simulink model "Microgrid_PV_WG_Bat_EV_j_22b"  (R2022b)
settings: Solver=VariableStepAuto  StartTime=0.0  StopTime=1  RelTol=1e-3
undefined symbols (not defined in the file or in its folder): Acid, Ion, Lead, Lithium
libraries: slpidlib x35, spsabctodq0Lib x23, spsSeriesRLCBranchLib x19, spsCurrentMeasurementLib x13, spsVoltageMeasurementLib x11, spsThreePhaseVIMeasurementLib x10, spsPLL3phLib x9, spsThreePhaseSeriesRLCBranchLib x9, spsPower3phInstantaneousLib x8, spsIGBTDiodeLib x8, spsUniversalBridgeLib x7, spsPWMGeneratorDCDCLib x6
(part 5 of 5)

== system Microgrid_PV_WG_Bat_EV_j_22b/DC//AC2/下垂控制/电压电流双闭环1 ==
  Vd_ref : Inport
  Vd : Inport  Port=2
  Vq_ref : Inport  Port=3
  Vq : Inport  Port=4
  Id : Inport  Port=5
  Iq : Inport  Port=6
  ILd : Inport  Port=7
  ILq : Inport  Port=8
  wt : Inport  Port=9
  Constant : Constant  Value=0
  Gain : Gain  Gain=2*pi*50*20e-6
  Gain1 : Gain  Gain=2*pi*50*20e-6
  Gain2 : Gain  Gain=2*pi*50
  Gain3 : Gain  Gain=2*pi*50
  L1 : Constant  Value=5e-3
  L2 : Constant  Value=5e-3
  Mux : Mux  Inputs=3
  PID Controller : slpidlib/PID Controller  Controller=PI  Form=Parallel  TimeDomain=Continuous-time  UseExternalTs=off  SampleTime=-1  IntegratorMethod=Forward Euler  FilterMethod=Forward Euler  ControllerParametersSource=internal  P=0.5  I=10  UseKiTs=off  D=0  N=100  UseFilter=on  TunerSelectOption=Transfer Function Based (PID Tuner App)  InitialConditionSource=internal  InitialConditionForIntegrator=0  InitialConditionForFilter=0  DifferentiatorICPrevScaledInput=0  ExternalReset=none  TrackingMode=off  Kt=1  LimitOutput=off  SatLimitsSource=internal  UpperSaturationLimit=inf  LowerSaturationLimit=-inf  LinearizeAsGain=on  AntiWindupMode=none  Kb=1  LimitIntegrator=off  UpperIntegratorSaturationLimit=inf  LowerIntegratorSaturationLimit=-inf  POutMin=[]  POutMax=[]  IOutMin=[]  IOutMax=[]  DOutMin=[]  DOutMax=[]  NOutMin=[]  NOutMax=[]  SumOutMin=[]  SumOutMax=[]  SaturationOutMin=[]  SaturationOutMax=[]  PParamMin=[]  PParamMax=[]  IParamMin=[]  IParamMax=[]  DParamMin=[]  DParamMax=[]  NParamMin=[]  NParamMax=[]  KbParamMin=[]  KbParamMax=[]  KtParamMin=[]  KtParamMax=[]  KbOutMin=[]  KbOutMax=[]  KtOutMin=[]  KtOutMax=[]  IntegratorOutMin=[]  IntegratorOutMax=[]  FilterOutMin=[]  FilterOutMax=[]  SumI1OutMin=[]  SumI1OutMax=[]  SumI2OutMin=[]  SumI2OutMax=[]  SumI3OutMin=[]  SumI3OutMax=[]  SumI4OutMin=[]  SumI4OutMax=[]  SumDOutMin=[]  SumDOutMax=[]  DifferentiatorOutMin=[]  DifferentiatorOutMax=[]  FilterDiffOutCoefMin=[]  FilterDiffOutCoefMax=[]  ReciprocalOutMin=[]  ReciprocalOutMax=[]  SumDenOutMin=[]  SumDenOutMax=[]  SumNumOutMin=[]  SumNumOutMax=[]  DivideOutMin=[]  DivideOutMax=[]  UdiffTsProdOutMin=[]  UdiffTsProdOutMax=[]  NTsProdOutMin=[]  NTsProdOutMax=[]  UintegralTsProdOutMin=[]  UintegralTsProdOutMax=[]  UngainTsProdOutMin=[]  UngainTsProdOutMax=[]  IntegratorContinuousStateAttributes=''  IntegratorStateMustResolveToSignalObject=off  IntegratorRTWStateStorageClass=Auto  FilterContinuousStateAttributes=''  FilterStateMustResolveToSignalObject=off  FilterRTWStateStorageClass=Auto  ParallelPVariant=InternalParameters  IdealPVariant=Disabled  IVariant=InternalParameters  DVariant=Disabled  IntegratorVariant=Continuous  SatVariant=Disabled  AWVariant=Passthrough  PCopyVariant=Disabled  TRVariant=Disabled  FdbkBlocksVariant=Forward  IdealPFdbkVariant=Disabled  SatFdbkVariant=Disabled  DerivativeFilterVariant=Disabled  NVariant=Disabled  NCopyVariant=Disabled_SignalSpec  FilterICVariant=Disabled  IntegratorICVariant=InternalICs  ExternalResetVariant=Disabled  TRSumVariant=Passthrough  SumFdbkVariant=Disabled  SumVariant=Sum_PI  TsampFilterVariant=InternalTs  TsampNgainVariant=Passthrough  TsampIntegralVariant=Disabled_SignalSpec  ExternalSaturationOutDataTypeStr=Inherit: Same as second input
  PID Controller1 : slpidlib/PID Controller  Controller=PI  Form=Parallel  TimeDomain=Continuous-time  UseExternalTs=off  SampleTime=-1  IntegratorMethod=Forward Euler  FilterMethod=Forward Euler  ControllerParametersSource=internal  P=0.5  I=10  UseKiTs=off  D=0  N=100  UseFilter=on  TunerSelectOption=Transfer Function Based (PID Tuner App)  InitialConditionSource=internal  InitialConditionForIntegrator=0  InitialConditionForFilter=0  DifferentiatorICPrevScaledInput=0  ExternalReset=none  TrackingMode=off  Kt=1  LimitOutput=off  SatLimitsSource=internal  UpperSaturationLimit=inf  LowerSaturationLimit=-inf  LinearizeAsGain=on  AntiWindupMode=none  Kb=1  LimitIntegrator=off  UpperIntegratorSaturationLimit=inf  LowerIntegratorSaturationLimit=-inf  POutMin=[]  POutMax=[]  IOutMin=[]  IOutMax=[]  DOutMin=[]  DOutMax=[]  NOutMin=[]  NOutMax=[]  SumOutMin=[]  SumOutMax=[]  SaturationOutMin=[]  SaturationOutMax=[]  PParamMin=[]  PParamMax=[]  IParamMin=[]  IParamMax=[]  DParamMin=[]  DParamMax=[]  NParamMin=[]  NParamMax=[]  KbParamMin=[]  KbParamMax=[]  KtParamMin=[]  KtParamMax=[]  KbOutMin=[]  KbOutMax=[]  KtOutMin=[]  KtOutMax=[]  IntegratorOutMin=[]  IntegratorOutMax=[]  FilterOutMin=[]  FilterOutMax=[]  SumI1OutMin=[]  SumI1OutMax=[]  SumI2OutMin=[]  SumI2OutMax=[]  SumI3OutMin=[]  SumI3OutMax=[]  SumI4OutMin=[]  SumI4OutMax=[]  SumDOutMin=[]  SumDOutMax=[]  DifferentiatorOutMin=[]  DifferentiatorOutMax=[]  FilterDiffOutCoefMin=[]  FilterDiffOutCoefMax=[]  ReciprocalOutMin=[]  ReciprocalOutMax=[]  SumDenOutMin=[]  SumDenOutMax=[]  SumNumOutMin=[]  SumNumOutMax=[]  DivideOutMin=[]  DivideOutMax=[]  UdiffTsProdOutMin=[]  UdiffTsProdOutMax=[]  NTsProdOutMin=[]  NTsProdOutMax=[]  UintegralTsProdOutMin=[]  UintegralTsProdOutMax=[]  UngainTsProdOutMin=[]  UngainTsProdOutMax=[]  IntegratorContinuousStateAttributes=''  IntegratorStateMustResolveToSignalObject=off  IntegratorRTWStateStorageClass=Auto  FilterContinuousStateAttributes=''  FilterStateMustResolveToSignalObject=off  FilterRTWStateStorageClass=Auto  ParallelPVariant=InternalParameters  IdealPVariant=Disabled  IVariant=InternalParameters  DVariant=Disabled  IntegratorVariant=Continuous  SatVariant=Disabled  AWVariant=Passthrough  PCopyVariant=Disabled  TRVariant=Disabled  FdbkBlocksVariant=Forward  IdealPFdbkVariant=Disabled  SatFdbkVariant=Disabled  DerivativeFilterVariant=Disabled  NVariant=Disabled  NCopyVariant=Disabled_SignalSpec  FilterICVariant=Disabled  IntegratorICVariant=InternalICs  ExternalResetVariant=Disabled  TRSumVariant=Passthrough  SumFdbkVariant=Disabled  SumVariant=Sum_PI  TsampFilterVariant=InternalTs  TsampNgainVariant=Passthrough  TsampIntegralVariant=Disabled_SignalSpec  ExternalSaturationOutDataTypeStr=Inherit: Same as second input
  PID Controller2 : slpidlib/PID Controller  Controller=PI  Form=Parallel  TimeDomain=Continuous-time  UseExternalTs=off  SampleTime=-1  IntegratorMethod=Forward Euler  FilterMethod=Forward Euler  ControllerParametersSource=internal  P=50  I=1000  UseKiTs=off  D=0  N=100  UseFilter=on  TunerSelectOption=Transfer Function Based (PID Tuner App)  InitialConditionSource=internal  InitialConditionForIntegrator=0  InitialConditionForFilter=0  DifferentiatorICPrevScaledInput=0  ExternalReset=none  TrackingMode=off  Kt=1  LimitOutput=off  SatLimitsSource=internal  UpperSaturationLimit=inf  LowerSaturationLimit=-inf  LinearizeAsGain=on  AntiWindupMode=none  Kb=1  LimitIntegrator=off  UpperIntegratorSaturationLimit=inf  LowerIntegratorSaturationLimit=-inf  POutMin=[]  POutMax=[]  IOutMin=[]  IOutMax=[]  DOutMin=[]  DOutMax=[]  NOutMin=[]  NOutMax=[]  SumOutMin=[]  SumOutMax=[]  SaturationOutMin=[]  SaturationOutMax=[]  PParamMin=[]  PParamMax=[]  IParamMin=[]  IParamMax=[]  DParamMin=[]  DParamMax=[]  NParamMin=[]  NParamMax=[]  KbParamMin=[]  KbParamMax=[]  KtParamMin=[]  KtParamMax=[]  KbOutMin=[]  KbOutMax=[]  KtOutMin=[]  KtOutMax=[]  IntegratorOutMin=[]  IntegratorOutMax=[]  FilterOutMin=[]  FilterOutMax=[]  SumI1OutMin=[]  SumI1OutMax=[]  SumI2OutMin=[]  SumI2OutMax=[]  SumI3OutMin=[]  SumI3OutMax=[]  SumI4OutMin=[]  SumI4OutMax=[]  SumDOutMin=[]  SumDOutMax=[]  DifferentiatorOutMin=[]  DifferentiatorOutMax=[]  FilterDiffOutCoefMin=[]  FilterDiffOutCoefMax=[]  ReciprocalOutMin=[]  ReciprocalOutMax=[]  SumDenOutMin=[]  SumDenOutMax=[]  SumNumOutMin=[]  SumNumOutMax=[]  DivideOutMin=[]  DivideOutMax=[]  UdiffTsProdOutMin=[]  UdiffTsProdOutMax=[]  NTsProdOutMin=[]  NTsProdOutMax=[]  UintegralTsProdOutMin=[]  UintegralTsProdOutMax=[]  UngainTsProdOutMin=[]  UngainTsProdOutMax=[]  IntegratorContinuousStateAttributes=''  IntegratorStateMustResolveToSignalObject=off  IntegratorRTWStateStorageClass=Auto  FilterContinuousStateAttributes=''  FilterStateMustResolveToSignalObject=off  FilterRTWStateStorageClass=Auto  ParallelPVariant=InternalParameters  IdealPVariant=Disabled  IVariant=InternalParameters  DVariant=Disabled  IntegratorVariant=Continuous  SatVariant=Disabled  AWVariant=Passthrough  PCopyVariant=Disabled  TRVariant=Disabled  FdbkBlocksVariant=Forward  IdealPFdbkVariant=Disabled  SatFdbkVariant=Disabled  DerivativeFilterVariant=Disabled  NVariant=Disabled  NCopyVariant=Disabled_SignalSpec  FilterICVariant=Disabled  IntegratorICVariant=InternalICs  ExternalResetVariant=Disabled  TRSumVariant=Passthrough  SumFdbkVariant=Disabled  SumVariant=Sum_PI  TsampFilterVariant=InternalTs  TsampNgainVariant=Passthrough  TsampIntegralVariant=Disabled_SignalSpec  ExternalSaturationOutDataTypeStr=Inherit: Same as second input
  PID Controller3 : slpidlib/PID Controller  Controller=PI  Form=Parallel  TimeDomain=Continuous-time  UseExternalTs=off  SampleTime=-1  IntegratorMethod=Forward Euler  FilterMethod=Forward Euler  ControllerParametersSource=internal  P=50  I=1000  UseKiTs=off  D=0  N=100  UseFilter=on  TunerSelectOption=Transfer Function Based (PID Tuner App)  InitialConditionSource=internal  InitialConditionForIntegrator=0  InitialConditionForFilter=0  DifferentiatorICPrevScaledInput=0  ExternalReset=none  TrackingMode=off  Kt=1  LimitOutput=off  SatLimitsSource=internal  UpperSaturationLimit=inf  LowerSaturationLimit=-inf  LinearizeAsGain=on  AntiWindupMode=none  Kb=1  LimitIntegrator=off  UpperIntegratorSaturationLimit=inf  LowerIntegratorSaturationLimit=-inf  POutMin=[]  POutMax=[]  IOutMin=[]  IOutMax=[]  DOutMin=[]  DOutMax=[]  NOutMin=[]  NOutMax=[]  SumOutMin=[]  SumOutMax=[]  SaturationOutMin=[]  SaturationOutMax=[]  PParamMin=[]  PParamMax=[]  IParamMin=[]  IParamMax=[]  DParamMin=[]  DParamMax=[]  NParamMin=[]  NParamMax=[]  KbParamMin=[]  KbParamMax=[]  KtParamMin=[]  KtParamMax=[]  KbOutMin=[]  KbOutMax=[]  KtOutMin=[]  KtOutMax=[]  IntegratorOutMin=[]  IntegratorOutMax=[]  FilterOutMin=[]  FilterOutMax=[]  SumI1OutMin=[]  SumI1OutMax=[]  SumI2OutMin=[]  SumI2OutMax=[]  SumI3OutMin=[]  SumI3OutMax=[]  SumI4OutMin=[]  SumI4OutMax=[]  SumDOutMin=[]  SumDOutMax=[]  DifferentiatorOutMin=[]  DifferentiatorOutMax=[]  FilterDiffOutCoefMin=[]  FilterDiffOutCoefMax=[]  ReciprocalOutMin=[]  ReciprocalOutMax=[]  SumDenOutMin=[]  SumDenOutMax=[]  SumNumOutMin=[]  SumNumOutMax=[]  DivideOutMin=[]  DivideOutMax=[]  UdiffTsProdOutMin=[]  UdiffTsProdOutMax=[]  NTsProdOutMin=[]  NTsProdOutMax=[]  UintegralTsProdOutMin=[]  UintegralTsProdOutMax=[]  UngainTsProdOutMin=[]  UngainTsProdOutMax=[]  IntegratorContinuousStateAttributes=''  IntegratorStateMustResolveToSignalObject=off  IntegratorRTWStateStorageClass=Auto  FilterContinuousStateAttributes=''  FilterStateMustResolveToSignalObject=off  FilterRTWStateStorageClass=Auto  ParallelPVariant=InternalParameters  IdealPVariant=Disabled  IVariant=InternalParameters  DVariant=Disabled  IntegratorVariant=Continuous  SatVariant=Disabled  AWVariant=Passthrough  PCopyVariant=Disabled  TRVariant=Disabled  FdbkBlocksVariant=Forward  IdealPFdbkVariant=Disabled  SatFdbkVariant=Disabled  DerivativeFilterVariant=Disabled  NVariant=Disabled  NCopyVariant=Disabled_SignalSpec  FilterICVariant=Disabled  IntegratorICVariant=InternalICs  ExternalResetVariant=Disabled  TRSumVariant=Passthrough  SumFdbkVariant=Disabled  SumVariant=Sum_PI  TsampFilterVariant=InternalTs  TsampNgainVariant=Passthrough  TsampIntegralVariant=Disabled_SignalSpec  ExternalSaturationOutDataTypeStr=Inherit: Same as second input
  PWM Generator (2-Level) : spsPWMGenerator2LevelLib/PWM Generator (2-Level)  ModulatorType=Three-phase bridge (6 pulses)  ModulatorMode=Unsynchronized  Fc=10e3  Pc=90  nF=27  MinMax="[ -1  1 ]"  SamplingTechnique=Natural  ModulatingSignals=off  m=0.8  Freq=60  Phase=0  Ts=0  ShowCarrierOutport=off
  Product1 : Product
  Product2 : Product
  Sum : Sum  Inputs=|+-
  Sum1 : Sum  Inputs=-+|
  Sum2 : Sum  Inputs=++-
  Sum3 : Sum  Inputs=+++
  Sum4 : Sum  Inputs=|+-
  Sum5 : Sum  Inputs=-+|
  Sum6 : Sum  Inputs=++-
  Sum7 : Sum  Inputs=+++
  dq0 to abc : spsdq0toabcLib/dq0 to abc  Alignment=90 degrees behind phase A axis
  PWM : Outport
  wires:
  Vd_ref/1 -> Sum/1
  Vd/1 -> Sum6/1, Sum/2, Gain/1
  Sum/1 -> PID Controller/1
  Sum1/1 -> PID Controller1/1
  Vq/1 -> Sum7/3, Gain1/1, Sum1/1
  PID Controller/1 -> Sum2/2
  PID Controller1/1 -> Sum3/2
  Gain1/1 -> Sum2/3
  Id/1 -> Sum2/1
  Sum2/1 -> Sum4/1  "ILd_ref"
  Sum3/1 -> Sum5/2  "ILq_ref"
  ILd/1 -> Gain2/1, Sum4/2
  Sum4/1 -> PID Controller2/1
  Sum5/1 -> PID Controller3/1
  PID Controller2/1 -> Sum6/2
  PID Controller3/1 -> Sum7/2
  Gain2/1 -> Product2/1
  L2/1 -> Product2/2
  Gain/1 -> Sum3/1
  Iq/1 -> Sum3/3
  Vq_ref/1 -> Sum1/2
  Product2/1 -> Sum7/1
  L1/1 -> Product1/1
  Gain3/1 -> Product1/2
  ILq/1 -> Gain3/1, Sum5/1
  Product1/1 -> Sum6/3
  Sum6/1 -> Mux/1  "ILd_ref"
  Sum7/1 -> Mux/2  "ILq_ref"
  Constant/1 -> Mux/3
  Mux/1 -> dq0 to abc/1
  wt/1 -> dq0 to abc/2
  dq0 to abc/1 -> PWM Generator (2-Level)/1
  PWM Generator (2-Level)/1 -> PWM/1

== system Microgrid_PV_WG_Bat_EV_j_22b/Subsystem4/Subsystem2/Subsystem ==
  电流 : Inport
  Fcn : Fcn  Expr=60000*8.3145*(273+T)*N*u(1)/(2*96485*P*101325*Uf_H2/100*x/100)
  Saturation : Saturate  UpperLimit=inf  LowerLimit=1
  流速 : Outport
  wires:
  电流/1 -> Fcn/1
  Fcn/1 -> Saturation/1
  Saturation/1 -> 流速/1

== system Microgrid_PV_WG_Bat_EV_j_22b/Subsystem4/Subsystem2/Subsystem1 ==
  电流 : Inport
  Fcn : Fcn  Expr=60000*8.3145*(273+T)*N*u(1)/(2*96485*P*101325*Uf_H2/100*x/100)
  Saturation : Saturate  UpperLimit=inf  LowerLimit=1
  流速 : Outport
  wires:
  Saturation/1 -> 流速/1
  Fcn/1 -> Saturation/1
  电流/1 -> Fcn/1

== system Microgrid_PV_WG_Bat_EV_j_22b/Subsystem4/Subsystem2/Subsystem2 ==
  Vd : Inport
  Vq : Inport  Port=2
  P : Inport  Port=3
  Q : Inport  Port=4
  Add10 : Sum  Inputs=+-
  Add5 : Sum
  Add6 : Sum
  Divide2 : Product  Inputs=*/
  Divide3 : Product  Inputs=/*
  Gain4 : Gain  Gain=2/3
  Gain5 : Gain  Gain=2/3
  Product{7..12} (6 alike) : Product
  Id_ref : Outport
  Iq_ref : Outport  Port=2
  wires:
  Add6/1 -> Divide3/1, Divide2/2
  Vd/1 -> Product9/2, Product9/1, Product7/1, Product10/1
  Add10/1 -> Gain5/1
  Vq/1 -> Product12/1, Product8/1, Product11/2, Product11/1
  Product9/1 -> Add6/1
  Gain4/1 -> Divide2/1
  Product7/1 -> Add5/1
  P/1 -> Product12/2, Product7/2
  Product12/1 -> Add10/1
  Gain5/1 -> Divide3/2
  Add5/1 -> Gain4/1
  Product10/1 -> Add10/2
  Product8/1 -> Add5/2
  Product11/1 -> Add6/2
  Q/1 -> Product10/2, Product8/2
  Divide3/1 -> Iq_ref/1  "Iq_ref"
  Divide2/1 -> Id_ref/1  "Id_ref"

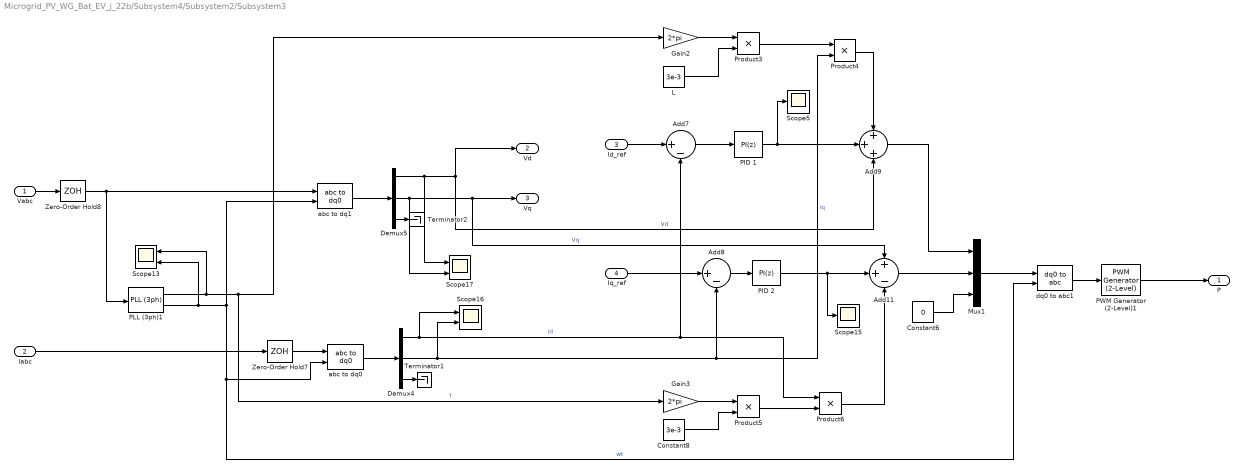
== system Microgrid_PV_WG_Bat_EV_j_22b/Subsystem4/Subsystem2/Subsystem3 ==
  Vabc : Inport
  Iabc : Inport  Port=2
  Id_ref : Inport  Port=3
  Iq_ref : Inport  Port=4
  Add11 : Sum  Inputs=++-
  Add7 : Sum  Inputs=|+-
  Add8 : Sum  Inputs=|+-
  Add9 : Sum  Inputs=+++
  Constant6 : Constant  Value=0
  Constant8 : Constant  Value=3e-3
  Demux4 : Demux  Outputs=3
  Demux5 : Demux  Outputs=3
  Gain2 : Gain  Gain=2*pi
  Gain3 : Gain  Gain=2*pi
  L : Constant  Value=3e-3
  Mux1 : Mux  Inputs=3
  PID 1 : slpidlib/PID Controller  Controller=PI  Form=Parallel  TimeDomain=Discrete-time  UseExternalTs=off  SampleTime=1e-5  IntegratorMethod=Forward Euler  FilterMethod=Forward Euler  ControllerParametersSource=internal  P=200  I=500  UseKiTs=off  D=0  N=100  UseFilter=on  TunerSelectOption=Transfer Function Based (PID Tuner App)  InitialConditionSource=internal  InitialConditionForIntegrator=0  InitialConditionForFilter=0  DifferentiatorICPrevScaledInput=0  ExternalReset=none  TrackingMode=off  Kt=1  LimitOutput=off  SatLimitsSource=internal  UpperSaturationLimit=0  LowerSaturationLimit=-860  LinearizeAsGain=on  AntiWindupMode=none  Kb=1  LimitIntegrator=off  UpperIntegratorSaturationLimit=inf  LowerIntegratorSaturationLimit=-inf  POutMin=[]  POutMax=[]  IOutMin=[]  IOutMax=[]  DOutMin=[]  DOutMax=[]  NOutMin=[]  NOutMax=[]  SumOutMin=[]  SumOutMax=[]  SaturationOutMin=[]  SaturationOutMax=[]  PParamMin=[]  PParamMax=[]  IParamMin=[]  IParamMax=[]  DParamMin=[]  DParamMax=[]  NParamMin=[]  NParamMax=[]  KbParamMin=[]  KbParamMax=[]  KtParamMin=[]  KtParamMax=[]  KbOutMin=[]  KbOutMax=[]  KtOutMin=[]  KtOutMax=[]  IntegratorOutMin=[]  IntegratorOutMax=[]  FilterOutMin=[]  FilterOutMax=[]  SumI1OutMin=[]  SumI1OutMax=[]  SumI2OutMin=[]  SumI2OutMax=[]  SumI3OutMin=[]  SumI3OutMax=[]  SumI4OutMin=[]  SumI4OutMax=[]  SumDOutMin=[]  SumDOutMax=[]  DifferentiatorOutMin=[]  DifferentiatorOutMax=[]  FilterDiffOutCoefMin=[]  FilterDiffOutCoefMax=[]  ReciprocalOutMin=[]  ReciprocalOutMax=[]  SumDenOutMin=[]  SumDenOutMax=[]  SumNumOutMin=[]  SumNumOutMax=[]  DivideOutMin=[]  DivideOutMax=[]  UdiffTsProdOutMin=[]  UdiffTsProdOutMax=[]  NTsProdOutMin=[]  NTsProdOutMax=[]  UintegralTsProdOutMin=[]  UintegralTsProdOutMax=[]  UngainTsProdOutMin=[]  UngainTsProdOutMax=[]  IntegratorContinuousStateAttributes=''  IntegratorStateMustResolveToSignalObject=off  IntegratorRTWStateStorageClass=Auto  FilterContinuousStateAttributes=''  FilterStateMustResolveToSignalObject=off  FilterRTWStateStorageClass=Auto  ParallelPVariant=InternalParameters  IdealPVariant=Disabled  IVariant=InternalParameters  DVariant=Disabled  IntegratorVariant=Discrete  SatVariant=Disabled  AWVariant=Passthrough  PCopyVariant=Disabled  TRVariant=Disabled  FdbkBlocksVariant=Forward  IdealPFdbkVariant=Disabled  SatFdbkVariant=Disabled  DerivativeFilterVariant=Disabled  NVariant=Disabled  NCopyVariant=Disabled_SignalSpec  FilterICVariant=Disabled  IntegratorICVariant=InternalICs  ExternalResetVariant=Disabled  TRSumVariant=Passthrough  SumFdbkVariant=Disabled  SumVariant=Sum_PI  TsampFilterVariant=InternalTs  TsampNgainVariant=Passthrough  TsampIntegralVariant=Disabled_SignalSpec  ExternalSaturationOutDataTypeStr=Inherit: Same as second input
  PID 2 : slpidlib/PID Controller  Controller=PI  Form=Parallel  TimeDomain=Discrete-time  UseExternalTs=off  SampleTime=1e-5  IntegratorMethod=Forward Euler  FilterMethod=Forward Euler  ControllerParametersSource=internal  P=200  I=500  UseKiTs=off  D=0  N=100  UseFilter=on  TunerSelectOption=Transfer Function Based (PID Tuner App)  InitialConditionSource=internal  InitialConditionForIntegrator=0  InitialConditionForFilter=0  DifferentiatorICPrevScaledInput=0  ExternalReset=none  TrackingMode=off  Kt=1  LimitOutput=off  SatLimitsSource=internal  UpperSaturationLimit=400  LowerSaturationLimit=-300  LinearizeAsGain=on  AntiWindupMode=none  Kb=1  LimitIntegrator=off  UpperIntegratorSaturationLimit=inf  LowerIntegratorSaturationLimit=-inf  POutMin=[]  POutMax=[]  IOutMin=[]  IOutMax=[]  DOutMin=[]  DOutMax=[]  NOutMin=[]  NOutMax=[]  SumOutMin=[]  SumOutMax=[]  SaturationOutMin=[]  SaturationOutMax=[]  PParamMin=[]  PParamMax=[]  IParamMin=[]  IParamMax=[]  DParamMin=[]  DParamMax=[]  NParamMin=[]  NParamMax=[]  KbParamMin=[]  KbParamMax=[]  KtParamMin=[]  KtParamMax=[]  KbOutMin=[]  KbOutMax=[]  KtOutMin=[]  KtOutMax=[]  IntegratorOutMin=[]  IntegratorOutMax=[]  FilterOutMin=[]  FilterOutMax=[]  SumI1OutMin=[]  SumI1OutMax=[]  SumI2OutMin=[]  SumI2OutMax=[]  SumI3OutMin=[]  SumI3OutMax=[]  SumI4OutMin=[]  SumI4OutMax=[]  SumDOutMin=[]  SumDOutMax=[]  DifferentiatorOutMin=[]  DifferentiatorOutMax=[]  FilterDiffOutCoefMin=[]  FilterDiffOutCoefMax=[]  ReciprocalOutMin=[]  ReciprocalOutMax=[]  SumDenOutMin=[]  SumDenOutMax=[]  SumNumOutMin=[]  SumNumOutMax=[]  DivideOutMin=[]  DivideOutMax=[]  UdiffTsProdOutMin=[]  UdiffTsProdOutMax=[]  NTsProdOutMin=[]  NTsProdOutMax=[]  UintegralTsProdOutMin=[]  UintegralTsProdOutMax=[]  UngainTsProdOutMin=[]  UngainTsProdOutMax=[]  IntegratorContinuousStateAttributes=''  IntegratorStateMustResolveToSignalObject=off  IntegratorRTWStateStorageClass=Auto  FilterContinuousStateAttributes=''  FilterStateMustResolveToSignalObject=off  FilterRTWStateStorageClass=Auto  ParallelPVariant=InternalParameters  IdealPVariant=Disabled  IVariant=InternalParameters  DVariant=Disabled  IntegratorVariant=Discrete  SatVariant=Disabled  AWVariant=Passthrough  PCopyVariant=Disabled  TRVariant=Disabled  FdbkBlocksVariant=Forward  IdealPFdbkVariant=Disabled  SatFdbkVariant=Disabled  DerivativeFilterVariant=Disabled  NVariant=Disabled  NCopyVariant=Disabled_SignalSpec  FilterICVariant=Disabled  IntegratorICVariant=InternalICs  ExternalResetVariant=Disabled  TRSumVariant=Passthrough  SumFdbkVariant=Disabled  SumVariant=Sum_PI  TsampFilterVariant=InternalTs  TsampNgainVariant=Passthrough  TsampIntegralVariant=Disabled_SignalSpec  ExternalSaturationOutDataTypeStr=Inherit: Same as second input
  PLL (3ph)1 : spsPLL3phLib/PLL (3ph)  Fmin=45  Par_Init=[0, 50]  ParK=[180, 3200, 1]  TcD=1e-4  MaxRateChangeFreq=12  FilterCutOffFreq=25  Ts=0  AGC=on
  PWM Generator (2-Level)1 : spsPWMGenerator2LevelLib/PWM Generator (2-Level)  ModulatorType=Three-phase bridge (6 pulses)  ModulatorMode=Unsynchronized  Fc=10000  Pc=90  nF=27  MinMax="[ -1  1 ]"  SamplingTechnique=Natural  ModulatingSignals=off  m=0.8  Freq=60  Phase=0  Ts=0  ShowCarrierOutport=off
  Product{3..6} (4 alike) : Product
  Scope13 : Scope  NumInputPorts=2
  Scope15 : Scope
  Scope16 : Scope  NumInputPorts=2
  Scope17 : Scope  NumInputPorts=2
  Scope5 : Scope
  Terminator1 : Terminator
  Terminator2 : Terminator
  Zero-Order Hold7 : ZeroOrderHold  SampleTime=1e-5
  Zero-Order Hold8 : ZeroOrderHold  SampleTime=1e-5
  abc to dq0 : spsabctodq0Lib/abc to dq0  Alignment=90 degrees behind phase A axis
  abc to dq1 : spsabctodq0Lib/abc to dq0  Alignment=90 degrees behind phase A axis
  dq0 to abc1 : spsdq0toabcLib/dq0 to abc  Alignment=90 degrees behind phase A axis
  P : Outport
  Vd : Outport  Port=2
  Vq : Outport  Port=3
  wires:
  Product6/1 -> Add11/3
  Gain2/1 -> Product3/1
  Add7/1 -> PID 1/1
  Constant8/1 -> Product5/2
  Add8/1 -> PID 2/1
  Product5/1 -> Product6/2
  Demux5/2 -> Vq/1, Add11/1, Scope17/2  "Vq"
  PLL (3ph)1/2 -> abc to dq1/2, abc to dq0/2, dq0 to abc1/2, Scope13/2  "wt"
  L/1 -> Product3/2
  Add11/1 -> Mux1/2
  PID 1/1 -> Scope5/1, Add9/2
  Mux1/1 -> dq0 to abc1/1
  Product4/1 -> Add9/1
  PID 2/1 -> Scope15/1, Add11/2
  Demux5/1 -> Vd/1, Add9/3, Scope17/1  "Vd"
  Constant6/1 -> Mux1/3
  Demux4/1 -> Scope16/1, Product6/1, Add7/2  "id"
  Product3/1 -> Product4/1
  Demux4/2 -> Add8/2, Product4/2, Scope16/2  "iq"
  abc to dq1/1 -> Demux5/1
  abc to dq0/1 -> Demux4/1
  Gain3/1 -> Product5/1
  Id_ref/1 -> Add7/1
  Demux4/3 -> Terminator1/1
  Zero-Order Hold8/1 -> abc to dq1/1, PLL (3ph)1/1
  Add9/1 -> Mux1/1
  Zero-Order Hold7/1 -> abc to dq0/1
  Demux5/3 -> Terminator2/1
  dq0 to abc1/1 -> PWM Generator (2-Level)1/1
  Iq_ref/1 -> Add8/1
  PLL (3ph)1/1 -> Gain2/1, Gain3/1, Scope13/1  "f"
  PWM Generator (2-Level)1/1 -> P/1
  Iabc/1 -> Zero-Order Hold7/1
  Vabc/1 -> Zero-Order Hold8/1

== system Microgrid_PV_WG_Bat_EV_j_22b/充电桩/恒流恒压充电/恒压 ==
  V : Inport
  Enable : EnablePort
  Constant3 : Constant  Value=500
  PID Controller1 : slpidlib/PID Controller  Controller=PID  Form=Parallel  TimeDomain=Discrete-time  UseExternalTs=off  SampleTime=1e-5  IntegratorMethod=Forward Euler  FilterMethod=Forward Euler  ControllerParametersSource=internal  P=50  I=50  UseKiTs=off  D=0  N=100  UseFilter=on  TunerSelectOption=Transfer Function Based (PID Tuner App)  InitialConditionSource=internal  InitialConditionForIntegrator=0  InitialConditionForFilter=0  DifferentiatorICPrevScaledInput=0  ExternalReset=none  TrackingMode=off  Kt=1  LimitOutput=off  SatLimitsSource=internal  UpperSaturationLimit=inf  LowerSaturationLimit=-inf  LinearizeAsGain=on  AntiWindupMode=none  Kb=1  LimitIntegrator=off  UpperIntegratorSaturationLimit=inf  LowerIntegratorSaturationLimit=-inf  POutMin=[]  POutMax=[]  IOutMin=[]  IOutMax=[]  DOutMin=[]  DOutMax=[]  NOutMin=[]  NOutMax=[]  SumOutMin=[]  SumOutMax=[]  SaturationOutMin=[]  SaturationOutMax=[]  PParamMin=[]  PParamMax=[]  IParamMin=[]  IParamMax=[]  DParamMin=[]  DParamMax=[]  NParamMin=[]  NParamMax=[]  KbParamMin=[]  KbParamMax=[]  KtParamMin=[]  KtParamMax=[]  KbOutMin=[]  KbOutMax=[]  KtOutMin=[]  KtOutMax=[]  IntegratorOutMin=[]  IntegratorOutMax=[]  FilterOutMin=[]  FilterOutMax=[]  SumI1OutMin=[]  SumI1OutMax=[]  SumI2OutMin=[]  SumI2OutMax=[]  SumI3OutMin=[]  SumI3OutMax=[]  SumI4OutMin=[]  SumI4OutMax=[]  SumDOutMin=[]  SumDOutMax=[]  DifferentiatorOutMin=[]  DifferentiatorOutMax=[]  FilterDiffOutCoefMin=[]  FilterDiffOutCoefMax=[]  ReciprocalOutMin=[]  ReciprocalOutMax=[]  SumDenOutMin=[]  SumDenOutMax=[]  SumNumOutMin=[]  SumNumOutMax=[]  DivideOutMin=[]  DivideOutMax=[]  UdiffTsProdOutMin=[]  UdiffTsProdOutMax=[]  NTsProdOutMin=[]  NTsProdOutMax=[]  UintegralTsProdOutMin=[]  UintegralTsProdOutMax=[]  UngainTsProdOutMin=[]  UngainTsProdOutMax=[]  IntegratorContinuousStateAttributes=''  IntegratorStateMustResolveToSignalObject=off  IntegratorRTWStateStorageClass=Auto  FilterContinuousStateAttributes=''  FilterStateMustResolveToSignalObject=off  FilterRTWStateStorageClass=Auto  ParallelPVariant=InternalParameters  IdealPVariant=Disabled  IVariant=InternalParameters  DVariant=InternalParameters  IntegratorVariant=Discrete  SatVariant=Disabled  AWVariant=Passthrough  PCopyVariant=Disabled  TRVariant=Disabled  FdbkBlocksVariant=Forward  IdealPFdbkVariant=Disabled  SatFdbkVariant=Disabled  DerivativeFilterVariant=ForwardEulerFilter  NVariant=InternalParameters  NCopyVariant=Disabled  FilterICVariant=InternalICsFilter  IntegratorICVariant=InternalICs  ExternalResetVariant=Disabled  TRSumVariant=Passthrough  SumFdbkVariant=Disabled  SumVariant=Sum_PID  TsampFilterVariant=InternalTs  TsampNgainVariant=Passthrough  TsampIntegralVariant=Disabled_SignalSpec  ExternalSaturationOutDataTypeStr=Inherit: Same as second input
  Sum3 : Sum  Inputs=|-+
  I_out : Outport
  wires:
  V/1 -> Sum3/1
  Constant3/1 -> Sum3/2
  Sum3/1 -> PID Controller1/1
  PID Controller1/1 -> I_out/1

== system Microgrid_PV_WG_Bat_EV_j_22b/充电桩/恒流恒压充电/恒流 ==
  I : Inport
  Enable : EnablePort
  Constant3 : Constant  Value=150
  PID Controller1 : slpidlib/PID Controller  Controller=PID  Form=Parallel  TimeDomain=Discrete-time  UseExternalTs=off  SampleTime=1e-5  IntegratorMethod=Forward Euler  FilterMethod=Forward Euler  ControllerParametersSource=internal  P=0.005  I=0.1  UseKiTs=off  D=0  N=100  UseFilter=on  TunerSelectOption=Transfer Function Based (PID Tuner App)  InitialConditionSource=internal  InitialConditionForIntegrator=0  InitialConditionForFilter=0  DifferentiatorICPrevScaledInput=0  ExternalReset=none  TrackingMode=off  Kt=1  LimitOutput=off  SatLimitsSource=internal  UpperSaturationLimit=inf  LowerSaturationLimit=-inf  LinearizeAsGain=on  AntiWindupMode=none  Kb=1  LimitIntegrator=off  UpperIntegratorSaturationLimit=inf  LowerIntegratorSaturationLimit=-inf  POutMin=[]  POutMax=[]  IOutMin=[]  IOutMax=[]  DOutMin=[]  DOutMax=[]  NOutMin=[]  NOutMax=[]  SumOutMin=[]  SumOutMax=[]  SaturationOutMin=[]  SaturationOutMax=[]  PParamMin=[]  PParamMax=[]  IParamMin=[]  IParamMax=[]  DParamMin=[]  DParamMax=[]  NParamMin=[]  NParamMax=[]  KbParamMin=[]  KbParamMax=[]  KtParamMin=[]  KtParamMax=[]  KbOutMin=[]  KbOutMax=[]  KtOutMin=[]  KtOutMax=[]  IntegratorOutMin=[]  IntegratorOutMax=[]  FilterOutMin=[]  FilterOutMax=[]  SumI1OutMin=[]  SumI1OutMax=[]  SumI2OutMin=[]  SumI2OutMax=[]  SumI3OutMin=[]  SumI3OutMax=[]  SumI4OutMin=[]  SumI4OutMax=[]  SumDOutMin=[]  SumDOutMax=[]  DifferentiatorOutMin=[]  DifferentiatorOutMax=[]  FilterDiffOutCoefMin=[]  FilterDiffOutCoefMax=[]  ReciprocalOutMin=[]  ReciprocalOutMax=[]  SumDenOutMin=[]  SumDenOutMax=[]  SumNumOutMin=[]  SumNumOutMax=[]  DivideOutMin=[]  DivideOutMax=[]  UdiffTsProdOutMin=[]  UdiffTsProdOutMax=[]  NTsProdOutMin=[]  NTsProdOutMax=[]  UintegralTsProdOutMin=[]  UintegralTsProdOutMax=[]  UngainTsProdOutMin=[]  UngainTsProdOutMax=[]  IntegratorContinuousStateAttributes=''  IntegratorStateMustResolveToSignalObject=off  IntegratorRTWStateStorageClass=Auto  FilterContinuousStateAttributes=''  FilterStateMustResolveToSignalObject=off  FilterRTWStateStorageClass=Auto  ParallelPVariant=InternalParameters  IdealPVariant=Disabled  IVariant=InternalParameters  DVariant=InternalParameters  IntegratorVariant=Discrete  SatVariant=Disabled  AWVariant=Passthrough  PCopyVariant=Disabled  TRVariant=Disabled  FdbkBlocksVariant=Forward  IdealPFdbkVariant=Disabled  SatFdbkVariant=Disabled  DerivativeFilterVariant=ForwardEulerFilter  NVariant=InternalParameters  NCopyVariant=Disabled  FilterICVariant=InternalICsFilter  IntegratorICVariant=InternalICs  ExternalResetVariant=Disabled  TRSumVariant=Passthrough  SumFdbkVariant=Disabled  SumVariant=Sum_PID  TsampFilterVariant=InternalTs  TsampNgainVariant=Passthrough  TsampIntegralVariant=Disabled_SignalSpec  ExternalSaturationOutDataTypeStr=Inherit: Same as second input
  Scope : Scope
  Sum3 : Sum  Inputs=|-+
  Zero-Order Hold : ZeroOrderHold  SampleTime=0.002
  I_out : Outport
  wires:
  Zero-Order Hold/1 -> Sum3/1
  I/1 -> Zero-Order Hold/1
  Constant3/1 -> Sum3/2
  PID Controller1/1 -> I_out/1
  Sum3/1 -> PID Controller1/1, Scope/1

== matlab function Microgrid_PV_WG_Bat_EV_j_22b/WindLog ==
  data: Vabc input; Iabc input; t input; Tstop input
function logPQsignals(Vabc, Iabc, t, Tstop)
% 适用于单个模块：记录Vabc/Iabc/P/Q/时间，并统一存入结构体

persistent P_log Q_log Va_log Vb_log Vc_log Ia_log Ib_log Ic_log time_log

if isempty(P_log)
    P_log = [];
    Q_log = [];
    Va_log = []; Vb_log = []; Vc_log = [];
    Ia_log = []; Ib_log = []; Ic_log = [];
    time_log = [];
end

% 拆解三相
Va = Vabc(1); Vb = Vabc(2); Vc = Vabc(3);
Ia = Iabc(1); Ib = Iabc(2); Ic = Iabc(3);

% 功率计算
P = Va * Ia + Vb * Ib + Vc * Ic;
Q = (Va*(Ib - Ic) + Vb*(Ic - Ia) + Vc*(Ia - Ib)) / sqrt(3);

% 每步记录
P_log(end+1) = P;
Q_log(end+1) = Q;
Va_log(end+1) = Va; Vb_log(end+1) = Vb; Vc_log(end+1) = Vc;
Ia_log(end+1) = Ia; Ib_log(end+1) = Ib; Ic_log(end+1) = Ic;
time_log(end+1) = t;

% 仿真结束保存结构体（!!! 只修改这一行结构体名字 !!!）
if abs(t - Tstop) < 1e-6
    ModuleLog.P = P_log;
    ModuleLog.Q = Q_log;
    ModuleLog.Va = Va_log;
    ModuleLog.Vb = Vb_log;
    ModuleLog.Vc = Vc_log;
    ModuleLog.Ia = Ia_log;
    ModuleLog.Ib = Ib_log;
    ModuleLog.Ic = Ic_log;
    ModuleLog.time = time_log;

    assignin('base', 'WindLog', ModuleLog);  % 👈 这里改成模块名
end

== matlab function Microgrid_PV_WG_Bat_EV_j_22b/PELLog ==
  data: Vabc input; Iabc input; t input; Tstop input
function logPQsignals(Vabc, Iabc, t, Tstop)
% 适用于单个模块：记录Vabc/Iabc/P/Q/时间，并统一存入结构体

persistent P_log Q_log Va_log Vb_log Vc_log Ia_log Ib_log Ic_log time_log

if isempty(P_log)
    P_log = [];
    Q_log = [];
    Va_log = []; Vb_log = []; Vc_log = [];
    Ia_log = []; Ib_log = []; Ic_log = [];
    time_log = [];
end

% 拆解三相
Va = Vabc(1); Vb = Vabc(2); Vc = Vabc(3);
Ia = Iabc(1); Ib = Iabc(2); Ic = Iabc(3);

% 功率计算
P = Va * Ia + Vb * Ib + Vc * Ic;
Q = (Va*(Ib - Ic) + Vb*(Ic - Ia) + Vc*(Ia - Ib)) / sqrt(3);

% 每步记录
P_log(end+1) = P;
Q_log(end+1) = Q;
Va_log(end+1) = Va; Vb_log(end+1) = Vb; Vc_log(end+1) = Vc;
Ia_log(end+1) = Ia; Ib_log(end+1) = Ib; Ic_log(end+1) = Ic;
time_log(end+1) = t;

% 仿真结束保存结构体（!!! 只修改这一行结构体名字 !!!）
if abs(t - Tstop) < 1e-6
    ModuleLog.P = P_log;
    ModuleLog.Q = Q_log;
    ModuleLog.Va = Va_log;
    ModuleLog.Vb = Vb_log;
    ModuleLog.Vc = Vc_log;
    ModuleLog.Ia = Ia_log;
    ModuleLog.Ib = Ib_log;
    ModuleLog.Ic = Ic_log;
    ModuleLog.time = time_log;

    assignin('base', 'PELLog', ModuleLog);  % 👈 这里改成模块名
end

== matlab function Microgrid_PV_WG_Bat_EV_j_22b/EVLog ==
  data: Vabc input; Iabc input; t input; Tstop input
function logPQsignals(Vabc, Iabc, t, Tstop)
% 适用于单个模块：记录Vabc/Iabc/P/Q/时间，并统一存入结构体

persistent P_log Q_log Va_log Vb_log Vc_log Ia_log Ib_log Ic_log time_log

if isempty(P_log)
    P_log = [];
    Q_log = [];
    Va_log = []; Vb_log = []; Vc_log = [];
    Ia_log = []; Ib_log = []; Ic_log = [];
    time_log = [];
end

% 拆解三相
Va = Vabc(1); Vb = Vabc(2); Vc = Vabc(3);
Ia = Iabc(1); Ib = Iabc(2); Ic = Iabc(3);

% 功率计算
P = Va * Ia + Vb * Ib + Vc * Ic;
Q = (Va*(Ib - Ic) + Vb*(Ic - Ia) + Vc*(Ia - Ib)) / sqrt(3);

% 每步记录
P_log(end+1) = P;
Q_log(end+1) = Q;
Va_log(end+1) = Va; Vb_log(end+1) = Vb; Vc_log(end+1) = Vc;
Ia_log(end+1) = Ia; Ib_log(end+1) = Ib; Ic_log(end+1) = Ic;
time_log(end+1) = t;

% 仿真结束保存结构体（!!! 只修改这一行结构体名字 !!!）
if abs(t - Tstop) < 1e-6
    ModuleLog.P = P_log;
    ModuleLog.Q = Q_log;
    ModuleLog.Va = Va_log;
    ModuleLog.Vb = Vb_log;
    ModuleLog.Vc = Vc_log;
    ModuleLog.Ia = Ia_log;
    ModuleLog.Ib = Ib_log;
    ModuleLog.Ic = Ic_log;
    ModuleLog.time = time_log;

    assignin('base', 'EVLog', ModuleLog);  % 👈 这里改成模块名
end

== matlab function Microgrid_PV_WG_Bat_EV_j_22b/脱网PCC点功率调节 ==
  settings: updateMethod=DISCRETE
  data: ModeSwitch input; t_now input; t_sync input; theta_micro input; theta_grid input; f_grid input; I_Grid input; P_bat input; P_PEL input; PLoad input; P_bat_out output; P_Grid input; P_PEL_out output; P_Load_out output; Breaker_Grid output; InverterModeSwitch output; delta_theta_comp output; wrapped_phase_diff output
function [P_bat_out, P_PEL_out, P_Load_out, Breaker_Grid, InverterModeSwitch, delta_theta_comp, wrapped_phase_diff]  = ...
    microgridControl(ModeSwitch, t_now, t_sync, theta_micro, theta_grid, f_grid, I_Grid, ...
    P_bat, P_PEL, PLoad, P_Grid)

% microgridControl - 统一的微电网运行控制函数模块
% 输入:
%   ModeSwitch   - 模式信号（0：离网；1：并网）
%   t_now        - 当前仿真时间
%   t_sync       - 计划并网时间
%   theta_micro  - 微电网当前相位
%   theta_grid   - 大电网当前相位
%   f_grid       - 大电网频率
%   I_Grid       - 并网点电流
%   P_bat        - 当前蓄电池功率
%   P_PEL        - 当前电解槽功率
%   PLoad        - 当前负载功率
%   P_Grid       - 当前并网功率
%   t_PVChange   - 光照改变时刻
%   t_WindChange - 风速改变时刻
% 输出:
%   P_bat_out    - 调整后蓄电池功率
%   P_PEL_out    - 调整后电解槽功率
%   P_Load_out   - 调整后负载功率
%   Breaker_Grid - 并网断路器状态（0：断开；1：闭合）
%   InverterModeSwitch  - 蓄电池逆变器策略（0：VF；1：PQ）
%   delta_theta_comp - 相位补偿量（VF控制使用）
%   wrapped_phase_diff - 经过处理后的相位差（范围在 [-pi, pi]）

% -------- 持久变量定义 --------
persistent flag P_bat_mem P_PEL_mem last_adjust_time Breaker_control_flag

% 相位同步控制相关
persistent Kp_sync Ki_sync phase_error_integral last_t_now;
persistent PHASE_TOLERANCE SYNC_DELAY_TIME sync_conditions_met_start_time;

% 持久变量初始化
if isempty(flag)
    flag = 1;
end
if isempty(P_bat_mem)
    P_bat_mem = 50000;
end
if isempty(P_PEL_mem)
    P_PEL_mem = 1000;
end
if isempty(last_adjust_time)
    last_adjust_time = -1;
end
if isempty(Breaker_control_flag)
    Breaker_control_flag = 1;
end

% === 相位同步控制器特有持久变量初始化 ===
if isempty(Kp_sync)
    Kp_sync = 0.05;   % 相位同步PI控制器比例增益
    Ki_sync = 1.5;     % 相位同步PI控制器积分增益
    phase_error_integral = 0;
    last_t_now = 0;

    PHASE_TOLERANCE = deg2rad(5); % 相位差容许值 (5度)
    SYNC_DELAY_TIME = 0.1;        % 保持同步条件满足的持续时间

    sync_conditions_met_start_time = -inf;
end

% --- 输出变量的默认值 ---
P_bat_out = P_bat_mem;
P_PEL_out = P_PEL_mem;
P_Load_out = PLoad;
Breaker_Grid = 0;
InverterModeSwitch = 1; % 默认PQ控制
delta_theta_comp = 0;   % 默认相位补偿为0
wrapped_phase_diff = 0; % 默认初始化 wrapped_phase_diff 为 0

% --- 计算当前仿真步长 (dt) ---
dt = t_now - last_t_now;
if dt <= 0
    dt = 1e-6;
end
last_t_now = t_now;

% --- 局部变量初始化 ---
current_calculated_delta_theta_comp = 0;

% -------- 脱网模式 (ModeSwitch == 0) --------
if ModeSwitch == 0
    Breaker_Grid = 1;
    InverterModeSwitch = 1;

    % 计划性脱网功率调整逻辑
    P_Grid_target = 1000;
    adjust_step = 5000;
    adjust_interval = 0.001;
    if t_now >= t_sync
        if abs(P_Grid) > P_Grid_target
            if t_now - last_adjust_time >= adjust_interval
                delta_P = sign(P_Grid) * min(abs(P_Grid), adjust_step);
                P_bat_out = P_bat + delta_P;
                last_adjust_time = t_now;
            end
        else
            Breaker_control_flag = 0;
        end

        if (abs(I_Grid) < 1e-2 && Breaker_control_flag == 0)
            Breaker_Grid = 0;
            InverterModeSwitch = 0; % 切换VF
        end
    end

    % 非计划性脱网处理
    if (f_grid < 49.5 || f_grid > 50.5)
        Breaker_Grid = 0;
        flag = 0;
    end
    if (abs(I_Grid) < 1e-2 && flag == 0)
        InverterModeSwitch = 0; % 切换VF
    end

    % 确保离网模式下相位同步PI状态重置
    phase_error_integral = 0;
    sync_conditions_met_start_time = -inf;

% -------- 并网模式 (ModeSwitch == 1) --------
else
    Breaker_Grid = 0;
    InverterModeSwitch = 0; % 默认VF，等待同步

    if t_now >= t_sync
        % 相位差计算与处理
        raw_phase_diff = theta_grid - theta_micro;
        wrapped_phase_diff = mod(raw_phase_diff + pi, 2*pi) - pi; % 计算并赋值给输出

        % 相位同步PI控制器
        if Breaker_Grid == 0
            phase_error_integral = phase_error_integral + wrapped_phase_diff * dt;

            % 限制积分项
            integral_limit = pi / 2;
            if phase_error_integral > integral_limit
                phase_error_integral = integral_limit;
            elseif phase_error_integral < -integral_limit
                integral_limit = -integral_limit; % Corrected assignment bug: should assign to integral_limit, not itself
            end
            current_calculated_delta_theta_comp = Kp_sync * wrapped_phase_diff + Ki_sync * phase_error_integral;
        else % 如果已经并网
            current_calculated_delta_theta_comp = 0;
            phase_error_integral = 0;
        end

        % 并网条件判断 (仅判断相位差)
        if abs(wrapped_phase_diff) < PHASE_TOLERANCE
            if sync_conditions_met_start_time == -inf
                sync_conditions_met_start_time = t_now;
            end
            if (t_now - sync_conditions_met_start_time) >= SYNC_DELAY_TIME
                Breaker_Grid = 1; % 闭合断路器
                InverterModeSwitch = 1; % 切换PQ
            end
        else % 相位差超出容差
            sync_conditions_met_start_time = -inf;
            Breaker_Grid = 0; % 断路器保持断开
            InverterModeSwitch = 0; % 继续VF同步
        end

        % 最终确定输出 delta_theta_comp
        if Breaker_Grid == 0
            delta_theta_comp = current_calculated_delta_theta_comp;
        else
            delta_theta_comp = 0;
        end
    end
end

% -------- 更新持久变量 --------
P_bat_mem = P_bat_out;
P_PEL_mem = P_PEL_out;
end

== matlab function Microgrid_PV_WG_Bat_EV_j_22b/GridLog ==
  data: Vabc input; Iabc input; t input; Tstop input
function logPQsignals(Vabc, Iabc, t, Tstop)
% 适用于单个模块：记录Vabc/Iabc/P/Q/时间，并统一存入结构体

persistent P_log Q_log Va_log Vb_log Vc_log Ia_log Ib_log Ic_log time_log

if isempty(P_log)
    P_log = [];
    Q_log = [];
    Va_log = []; Vb_log = []; Vc_log = [];
    Ia_log = []; Ib_log = []; Ic_log = [];
    time_log = [];
end

% 拆解三相
Va = Vabc(1); Vb = Vabc(2); Vc = Vabc(3);
Ia = Iabc(1); Ib = Iabc(2); Ic = Iabc(3);

% 功率计算
P = Va * Ia + Vb * Ib + Vc * Ic;
Q = (Va*(Ib - Ic) + Vb*(Ic - Ia) + Vc*(Ia - Ib)) / sqrt(3);

% 每步记录
P_log(end+1) = P;
Q_log(end+1) = Q;
Va_log(end+1) = Va; Vb_log(end+1) = Vb; Vc_log(end+1) = Vc;
Ia_log(end+1) = Ia; Ib_log(end+1) = Ib; Ic_log(end+1) = Ic;
time_log(end+1) = t;

% 仿真结束保存结构体（!!! 只修改这一行结构体名字 !!!）
if abs(t - Tstop) < 1e-6
    ModuleLog.P = P_log;
    ModuleLog.Q = Q_log;
    ModuleLog.Va = Va_log;
    ModuleLog.Vb = Vb_log;
    ModuleLog.Vc = Vc_log;
    ModuleLog.Ia = Ia_log;
    ModuleLog.Ib = Ib_log;
    ModuleLog.Ic = Ic_log;
    ModuleLog.time = time_log;

    assignin('base', 'GridLog', ModuleLog);  % 👈 这里改成模块名
end

== matlab function Microgrid_PV_WG_Bat_EV_j_22b/Model_Control ==
  data: t_PVChange input; PV_Change output; t_WindChange input; Wind_Change output; t_now input; Change_enable input
function [PV_Change,Wind_Change] = fcn(t_PVChange,t_WindChange, t_now,Change_enable)
PV_Change=0;
Wind_Change=0;
if Change_enable==1
 if t_now > t_PVChange
     PV_Change=-400;
 end
 if t_now > t_WindChange
     Wind_Change=-3;
 end
else
    PV_Change=0;
    Wind_Change=0;
end

== matlab function Microgrid_PV_WG_Bat_EV_j_22b/BatteryLog ==
  data: Vabc input; Iabc input; t input; Tstop input
function logPQsignals(Vabc, Iabc, t, Tstop)
% 适用于单个模块：记录Vabc/Iabc/P/Q/时间，并统一存入结构体

persistent P_log Q_log Va_log Vb_log Vc_log Ia_log Ib_log Ic_log time_log

if isempty(P_log)
    P_log = [];
    Q_log = [];
    Va_log = []; Vb_log = []; Vc_log = [];
    Ia_log = []; Ib_log = []; Ic_log = [];
    time_log = [];
end

% 拆解三相
Va = Vabc(1); Vb = Vabc(2); Vc = Vabc(3);
Ia = Iabc(1); Ib = Iabc(2); Ic = Iabc(3);

% 功率计算
P = Va * Ia + Vb * Ib + Vc * Ic;
Q = (Va*(Ib - Ic) + Vb*(Ic - Ia) + Vc*(Ia - Ib)) / sqrt(3);

% 每步记录
P_log(end+1) = P;
Q_log(end+1) = Q;
Va_log(end+1) = Va; Vb_log(end+1) = Vb; Vc_log(end+1) = Vc;
Ia_log(end+1) = Ia; Ib_log(end+1) = Ib; Ic_log(end+1) = Ic;
time_log(end+1) = t;

% 仿真结束保存结构体（!!! 只修改这一行结构体名字 !!!）
if abs(t - Tstop) < 1e-6
    ModuleLog.P = P_log;
    ModuleLog.Q = Q_log;
    ModuleLog.Va = Va_log;
    ModuleLog.Vb = Vb_log;
    ModuleLog.Vc = Vc_log;
    ModuleLog.Ia = Ia_log;
    ModuleLog.Ib = Ib_log;
    ModuleLog.Ic = Ic_log;
    ModuleLog.time = time_log;

    assignin('base', 'BatteryLog', ModuleLog);  % 👈 这里改成模块名
end

== matlab function Microgrid_PV_WG_Bat_EV_j_22b/PVLog ==
  data: Vabc input; Iabc input; t input; Tstop input
function logPQsignals(Vabc, Iabc, t, Tstop)
% 适用于单个模块：记录Vabc/Iabc/P/Q/时间，并统一存入结构体

persistent P_log Q_log Va_log Vb_log Vc_log Ia_log Ib_log Ic_log time_log

if isempty(P_log)
    P_log = [];
    Q_log = [];
    Va_log = []; Vb_log = []; Vc_log = [];
    Ia_log = []; Ib_log = []; Ic_log = [];
    time_log = [];
end

% 拆解三相
Va = Vabc(1); Vb = Vabc(2); Vc = Vabc(3);
Ia = Iabc(1); Ib = Iabc(2); Ic = Iabc(3);

% 功率计算
P = Va * Ia + Vb * Ib + Vc * Ic;
Q = (Va*(Ib - Ic) + Vb*(Ic - Ia) + Vc*(Ia - Ib)) / sqrt(3);

% 每步记录
P_log(end+1) = P;
Q_log(end+1) = Q;
Va_log(end+1) = Va; Vb_log(end+1) = Vb; Vc_log(end+1) = Vc;
Ia_log(end+1) = Ia; Ib_log(end+1) = Ib; Ic_log(end+1) = Ic;
time_log(end+1) = t;

% 仿真结束保存结构体（!!! 只修改这一行结构体名字 !!!）
if abs(t - Tstop) < 1e-6
    ModuleLog.P = P_log;
    ModuleLog.Q = Q_log;
    ModuleLog.Va = Va_log;
    ModuleLog.Vb = Vb_log;
    ModuleLog.Vc = Vc_log;
    ModuleLog.Ia = Ia_log;
    ModuleLog.Ib = Ib_log;
    ModuleLog.Ic = Ic_log;
    ModuleLog.time = time_log;

    assignin('base', 'PVLog', ModuleLog);  % 👈 这里改成模块名
end

== matlab function Microgrid_PV_WG_Bat_EV_j_22b/LoadLog ==
  data: Vabc input; Iabc input; t input; Tstop input
function logPQsignals(Vabc, Iabc, t, Tstop)
% 适用于单个模块：记录Vabc/Iabc/P/Q/时间，并统一存入结构体

persistent P_log Q_log Va_log Vb_log Vc_log Ia_log Ib_log Ic_log time_log

if isempty(P_log)
    P_log = [];
    Q_log = [];
    Va_log = []; Vb_log = []; Vc_log = [];
    Ia_log = []; Ib_log = []; Ic_log = [];
    time_log = [];
end

% 拆解三相
Va = Vabc(1); Vb = Vabc(2); Vc = Vabc(3);
Ia = Iabc(1); Ib = Iabc(2); Ic = Iabc(3);

% 功率计算
P = Va * Ia + Vb * Ib + Vc * Ic;
Q = (Va*(Ib - Ic) + Vb*(Ic - Ia) + Vc*(Ia - Ib)) / sqrt(3);

% 每步记录
P_log(end+1) = P;
Q_log(end+1) = Q;
Va_log(end+1) = Va; Vb_log(end+1) = Vb; Vc_log(end+1) = Vc;
Ia_log(end+1) = Ia; Ib_log(end+1) = Ib; Ic_log(end+1) = Ic;
time_log(end+1) = t;

% 仿真结束保存结构体（!!! 只修改这一行结构体名字 !!!）
if abs(t - Tstop) < 1e-6
    ModuleLog.P = P_log;
    ModuleLog.Q = Q_log;
    ModuleLog.Va = Va_log;
    ModuleLog.Vb = Vb_log;
    ModuleLog.Vc = Vc_log;
    ModuleLog.Ia = Ia_log;
    ModuleLog.Ib = Ib_log;
    ModuleLog.Ic = Ic_log;
    ModuleLog.time = time_log;

    assignin('base', 'LoadLog', ModuleLog);  % 👈 这里改成模块名
end
